simulink model "hydrotwin_realtime"  (R2025b)
settings: Solver=FixedStepAuto  StartTime=0.0  StopTime=1814400  FixedStep=300  RelTol=1e-3
settings Model: Creator=furkan  LastModifiedBy=furkan

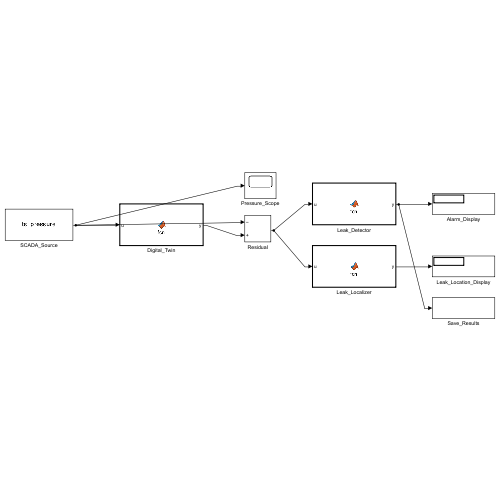
[thumbnail: Simulink's stored preview of the top-level diagram]
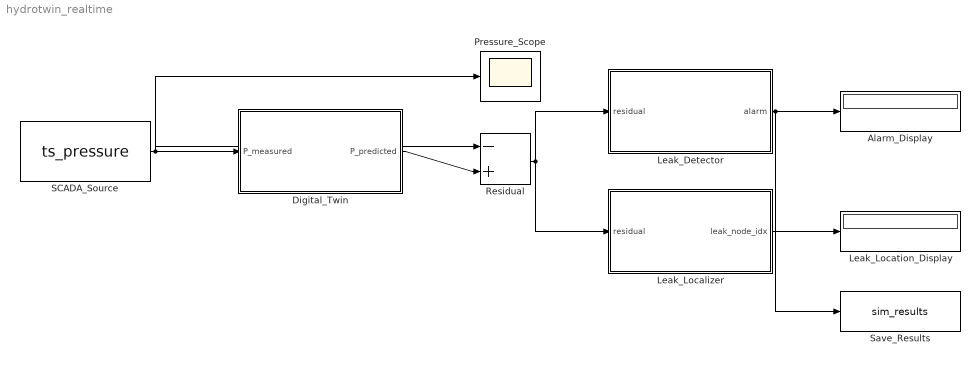
== system hydrotwin_realtime ==
  Alarm_Display : Display
  Digital_Twin : MATLAB Function  TreatAsAtomicUnit=on
  Leak_Detector : MATLAB Function  TreatAsAtomicUnit=on
  Leak_Localizer : MATLAB Function  TreatAsAtomicUnit=on
  Leak_Location_Display : Display
  Pressure_Scope : Scope
  Residual : Sum  Inputs=-+
  SCADA_Source : FromWorkspace  VariableName=ts_pressure
  Save_Results : ToWorkspace  VariableName=sim_results  SaveFormat=Timeseries  SampleTime=-1
  wires:
  SCADA_Source/1 -> Digital_Twin/1(P_measured), Residual/1, Pressure_Scope/1
  Digital_Twin/1(P_predicted) -> Residual/2
  Residual/1 -> Leak_Detector/1(residual), Leak_Localizer/1(residual)
  Leak_Detector/1(alarm) -> Alarm_Display/1, Save_Results/1
  Leak_Localizer/1(leak_node_idx) -> Leak_Location_Display/1

== matlab function hydrotwin_realtime/Digital_Twin ==
  data: P_measured input; P_predicted output
function P_predicted = Digital_Twin(P_measured)
%#codegen
% Plan C: model-driven nominal + online bias correction (ilk 24h)

persistent P_nom bias t_idx N_calib init

if isempty(init)
    data    = coder.load('digital_twin_data.mat');
    P_nom   = data.P_nominal_demo;
    bias    = zeros(33, 1);
    t_idx   = int32(0);
    N_calib = int32(288);
    init    = true;
end

t_idx = t_idx + 1;

ti = t_idx;
if ti > int32(size(P_nom, 1))
    ti = int32(size(P_nom, 1));
end

P_nom_now = P_nom(ti, :)';

if t_idx <= N_calib
    alpha = 1.0 / double(t_idx);
    bias  = bias * (1 - alpha) + (P_measured - P_nom_now) * alpha;
end

P_predicted = P_nom_now + bias;
end

== matlab function hydrotwin_realtime/Leak_Localizer ==
  data: residual input; leak_node_idx output
function leak_node_idx = Leak_Localizer(residual)
%#codegen
% Mantık:
%   1) İlk 288 sample (24h) kalibrasyon → 0
%   2) Adaptif threshold + 12 sample persistence → alarm tetiklendi
%   3) Alarm sonrası 288 sample (24h) bekle
%   4) Son 288 sample'ın ortalamasıyla LOCALIZE et + DONDUR

persistent S_norm last_idx threshold buffer t_idx N_calib N_window K counter alarm_t init

if isempty(init)
    data      = coder.load('digital_twin_data.mat');
    S_norm    = data.S_norm;
    threshold = data.threshold_adaptive;
    last_idx  = 0;
    N_window  = int32(288);
    buffer    = zeros(33, 288);
    t_idx     = int32(0);
    N_calib   = int32(288);
    K         = int32(12);
    counter   = int32(0);
    alarm_t   = int32(-1);
    init      = true;
end

t_idx = t_idx + 1;

% Sliding buffer
buffer(:, 1:end-1) = buffer(:, 2:end);
buffer(:, end)     = residual;

% (1) Kalibrasyon
if t_idx <= N_calib
    leak_node_idx = 0;
    return;
end

% (2) Alarm henüz tetiklenmediyse
if alarm_t < 0
    if norm(residual) > threshold
        counter = counter + 1;
        if counter >= K
            alarm_t = t_idx;
        end
    else
        counter = int32(0);
    end
    leak_node_idx = 0;
    return;
end

% (3 + 4) Alarm + 24h sonra LOCALIZE ve DONDUR
if last_idx == 0 && (t_idx - alarm_t) >= N_window
    r_avg = mean(buffer, 2);
    r     = r_avg / (norm(r_avg) + 1e-9);
    corr  = S_norm' * r;
    [~, idx] = max(corr);
    last_idx = double(idx);
end

leak_node_idx = last_idx;
end

== matlab function hydrotwin_realtime/Leak_Detector ==
  data: residual input; alarm output
function alarm = Leak_Detector(residual)
%#codegen
% Adaptif threshold + persistence: q95×1.3 üstünde 12 sample (1h) → alarm
% Latching: bir kere yandı mı söndürmez

persistent threshold K counter state t_idx N_calib init

if isempty(init)
    data      = coder.load('digital_twin_data.mat');
    threshold = data.threshold_adaptive;
    K         = int32(12);
    counter   = int32(0);
    state     = false;
    t_idx     = int32(0);
    N_calib   = int32(288);
    init      = true;
end

t_idx = t_idx + 1;

if t_idx <= N_calib
    alarm = 0;
    return;
end

if norm(residual) > threshold
    counter = counter + 1;
    if counter >= K
        state = true;
    end
else
    counter = int32(0);
end

alarm = double(state);
end
